simulink model "PoredjenjeLinNelin"  (R2018a)
settings: Solver=VariableStepAuto  StartTime=0.0  StopTime=30  RelTol=1e-3  EnableMultiTasking=on
values from neighbouring files (symbols this model uses):
  a11 = double(subs(diff(f1,wm),[wm id iq u1 mh],[wmn idn iqn u1n mhn]))    [Linearizacija.m]
  a12 = double(subs(diff(f1,id),[wm id iq u1 mh],[wmn idn iqn u1n mhn]))    [Linearizacija.m]
  a13 = double(subs(diff(f1,iq),[wm id iq u1 mh],[wmn idn iqn u1n mhn]))    [Linearizacija.m]
  a21 = double(subs(diff(f2,wm),[wm id iq u1 mh],[wmn idn iqn u1n mhn]))    [Linearizacija.m]
  a22 = double(subs(diff(f2,id),[wm id iq u1 mh],[wmn idn iqn u1n mhn]))    [Linearizacija.m]
  a23 = double(subs(diff(f2,iq),[wm id iq u1 mh],[wmn idn iqn u1n mhn]))    [Linearizacija.m]
  a31 = double(subs(diff(f3,wm),[wm id iq u1 mh],[wmn idn iqn u1n mhn]))    [Linearizacija.m]
  a32 = double(subs(diff(f3,id),[wm id iq u1 mh],[wmn idn iqn u1n mhn]))    [Linearizacija.m]
  a33 = double(subs(diff(f3,iq),[wm id iq u1 mh],[wmn idn iqn u1n mhn]))    [Linearizacija.m]
  b11 = double(subs(diff(f1,u1),[wm id iq u1 mh],[wmn idn iqn u1n mhn]))    [Linearizacija.m]
  b12 = double(subs(diff(f1,mh),[wm id iq u1 mh],[wmn idn iqn u1n mhn]))    [Linearizacija.m]
  b21 = double(subs(diff(f2,u1),[wm id iq u1 mh],[wmn idn iqn u1n mhn]))    [Linearizacija.m]
  b22 = double(subs(diff(f2,mh),[wm id iq u1 mh],[wmn idn iqn u1n mhn]))    [Linearizacija.m]
  b31 = double(subs(diff(f3,u1),[wm id iq u1 mh],[wmn idn iqn u1n mhn]))    [Linearizacija.m]
  b32 = double(subs(diff(f3,mh),[wm id iq u1 mh],[wmn idn iqn u1n mhn]))    [Linearizacija.m]
  Bv = 1.349*10^(-5)    (= 1.349e-05)    [Podaci.m]    (also in Podaci.mat)
  F0 = 0.1717    [Podaci.m]    (also in Podaci.mat)
  idn = Odgovor(2)    [nominale.m]
  iqn = Odgovor(3)    [nominale.m]
  J0 = 3.26*10^-3    (= 0.00326)    [Podaci.m]    (also in Podaci.mat)
  Ls = Ld    (= 0.03682)    [Podaci.m]    (also in Podaci.mat)
  m = 3    [Podaci.m]    (also in Podaci.mat)
  mhn = 0.3    [nominale.m]
  np = 2    [Podaci.m]    (also in Podaci.mat)
  Rs = 16.7    [Podaci.m]    (also in Podaci.mat)
  teta0 = 0    [Podaci.m]    (also in Podaci.mat)
  u1n = Odgovor(1)    [nominale.m]
  wmn = nn*pi/30    (= 314.159265359)    [nominale.m]
settings Model: Creator=Bane  LastModifiedBy=lakim
settings DataIOCC: LimitDataPoints=on
settings OptimizationCC: LifeSpan=inf
settings DebuggingCC: AllowSymbolicDim=off  SFUnexpectedBacktrackingDiag=warning  SFNoUnconditionalDefaultTransitionDiag=warning  SFExecutionAtInitializationDiag=none
settings ModelReferenceCC: PropagateSignalLabelsOutOfModel=off
settings CodeAppCC: StateflowObjectComments=on
settings GRTTargetCC: TargetLangStandard=C89/C90 (ANSI)
settings ConfigComp: CovMetricSettings=dw  CovHtmlReporting=on  CovSaveCumulativeToWorkspaceVar=on  CovSaveSingleToWorkspaceVar=on  CovExternalEMLEnable=off

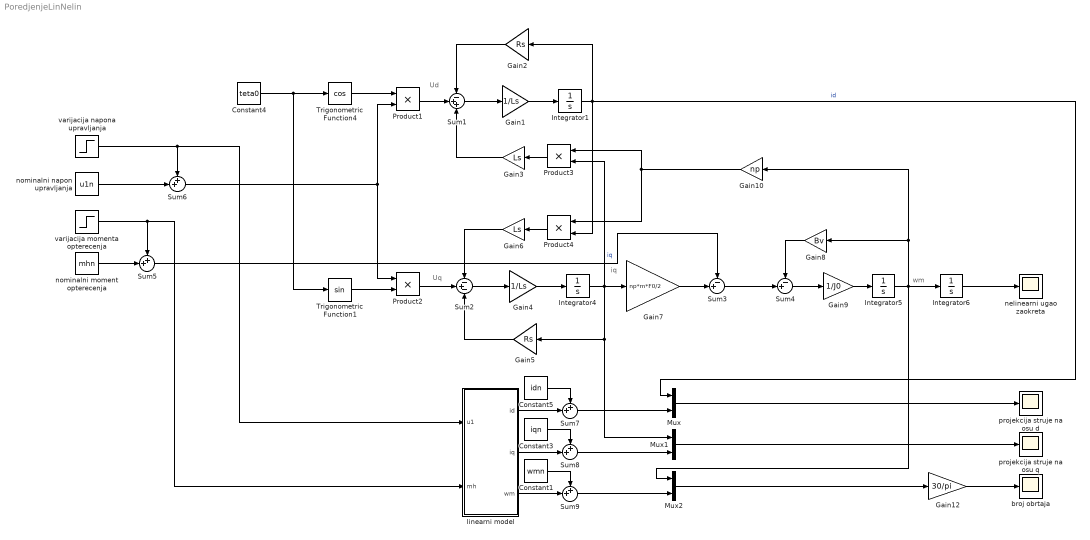
== system PoredjenjeLinNelin ==
  note: Uq
  note: iq
  note: Ud
  note: wm
  " broj obrtaja" : Scope
  Constant1 : Constant  Value=wmn
  Constant3 : Constant  Value=iqn
  Constant4 : Constant  Value=teta0
  Constant5 : Constant  Value=idn
  Gain1 : Gain  Gain=1/Ls
  Gain10 : Gain  Gain=np
  Gain12 : Gain  Gain=30/pi
  Gain2 : Gain  Gain=Rs
  Gain3 : Gain  Gain=Ls
  Gain4 : Gain  Gain=1/Ls
  Gain5 : Gain  Gain=Rs
  Gain6 : Gain  Gain=Ls
  Gain7 : Gain  Gain=np*m*F0/2
  Gain8 : Gain  Gain=Bv
  Gain9 : Gain  Gain=1/J0
  Integrator1 : Integrator  InitialCondition=idn
  Integrator4 : Integrator  InitialCondition=iqn
  Integrator5 : Integrator  InitialCondition=wmn
  Integrator6 : Integrator
  Mux : Mux  Inputs=2
  Mux1 : Mux  Inputs=2
  Mux2 : Mux  Inputs=2
  Product{1..4} (4 alike) : Product
  Sum1 : Sum  Inputs=-++
  Sum2 : Sum  Inputs=-+-
  Sum3 : Sum  Inputs=-+|
  Sum4 : Sum  Inputs=-+|
  Sum{5..9} (5 alike) : Sum  Inputs=++|
  Trigonometric Function1 : Trigonometry
  Trigonometric Function4 : Trigonometry  Operator=cos
  linearni model : Subsystem
  nelinearni ugao zaokreta : Scope
  nominalni moment opterecenja : Constant  Value=mhn
  nominalni napon upravljanja : Constant  Value=u1n
  projekcija struje na osu d : Scope
  projekcija struje na osu q : Scope
  "varijacija momenta opterecenja " : Step  Time=3  After=0.3  SampleTime=0
  varijacija napona upravljanja : Step  Time=0  After=0  SampleTime=0
  wires:
  Gain1/1 -> Integrator1/1
  Integrator1/1 -> Mux/1, Product4/2, Gain2/1  "id"
  Gain2/1 -> Sum1/1
  Sum1/1 -> Gain1/1
  Trigonometric Function1/1 -> Product2/2
  Trigonometric Function4/1 -> Product1/1
  Constant4/1 -> Trigonometric Function1/1, Trigonometric Function4/1
  Product1/1 -> Sum1/2
  Product3/1 -> Gain3/1
  Gain3/1 -> Sum1/3
  Gain4/1 -> Integrator4/1
  Integrator4/1 -> Mux1/1, Gain5/1, Gain7/1, Product3/2  "iq"
  Sum2/1 -> Gain4/1
  Product2/1 -> Sum2/2
  Product4/1 -> Gain6/1
  Gain6/1 -> Sum2/1
  Gain5/1 -> Sum2/3
  Gain9/1 -> Integrator5/1
  Integrator5/1 -> Mux2/1, Integrator6/1, Gain10/1, Gain8/1
  Sum4/1 -> Gain9/1
  Gain8/1 -> Sum4/1
  Gain10/1 -> Product4/1, Product3/1
  Integrator6/1 -> nelinearni ugao zaokreta/1
  Gain7/1 -> Sum3/2
  Sum3/1 -> Sum4/2
  nominalni moment opterecenja/1 -> Sum5/2
  Sum5/1 -> Sum3/1
  "varijacija momenta opterecenja "/1 -> linearni model/2(mh), Sum5/1
  Sum6/1 -> Product2/1, Product1/2
  nominalni napon upravljanja/1 -> Sum6/2
  varijacija napona upravljanja/1 -> Sum6/1, linearni model/1(u1)
  Mux/1 -> projekcija struje na osu d/1
  Mux2/1 -> Gain12/1
  linearni model/1(id) -> Sum7/2
  Sum7/1 -> Mux/2
  linearni model/2(iq) -> Sum8/2
  linearni model/3(wm) -> Sum9/2
  Sum9/1 -> Mux2/2
  Constant5/1 -> Sum7/1
  Constant3/1 -> Sum8/1
  Constant1/1 -> Sum9/1
  Gain12/1 -> " broj obrtaja"/1
  Mux1/1 -> projekcija struje na osu q/1
  Sum8/1 -> Mux1/2

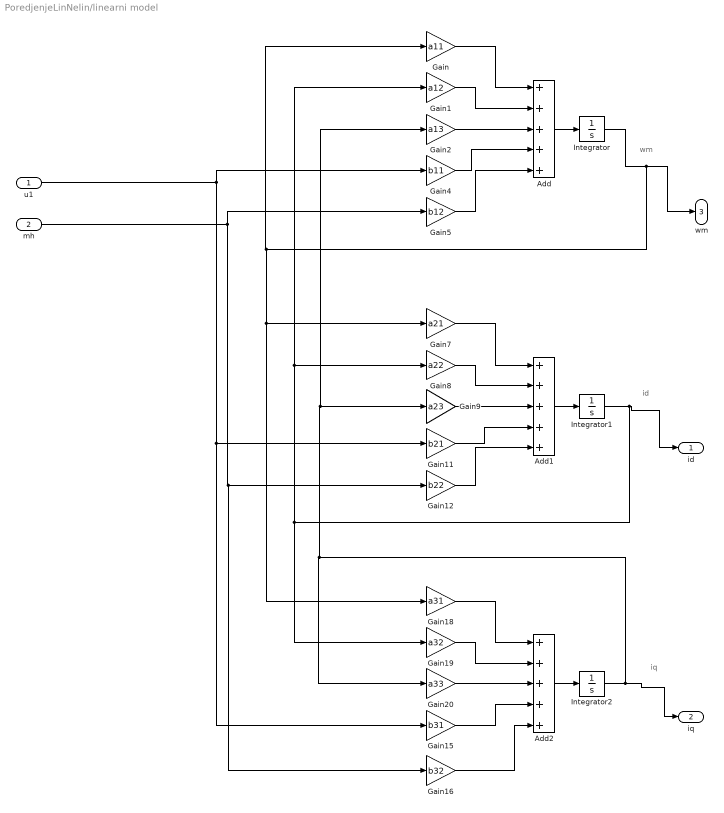
== system PoredjenjeLinNelin/linearni model ==
  note: wm
  note: iq
  note: id
  u1 : Inport
  mh : Inport  Port=2
  Add : Sum  Inputs=+++++
  Add1 : Sum  Inputs=+++++
  Add2 : Sum  Inputs=+++++
  Gain : Gain  Gain=a11
  Gain1 : Gain  Gain=a12
  Gain11 : Gain  Gain=b21
  Gain12 : Gain  Gain=b22
  Gain15 : Gain  Gain=b31
  Gain16 : Gain  Gain=b32
  Gain18 : Gain  Gain=a31
  Gain19 : Gain  Gain=a32
  Gain2 : Gain  Gain=a13
  Gain20 : Gain  Gain=a33
  Gain4 : Gain  Gain=b11
  Gain5 : Gain  Gain=b12
  Gain7 : Gain  Gain=a21
  Gain8 : Gain  Gain=a22
  Gain9 : Gain  Gain=a23
  Integrator : Integrator
  Integrator1 : Integrator
  Integrator2 : Integrator
  id : Outport  VectorParamsAs1DForOutWhenUnconnected=on
  iq : Outport  Port=2  VectorParamsAs1DForOutWhenUnconnected=on
  wm : Outport  Port=3  VectorParamsAs1DForOutWhenUnconnected=on
  wires:
  Gain4/1 -> Add/4
  Gain5/1 -> Add/5
  Gain18/1 -> Add2/1
  Gain2/1 -> Add/3
  Add2/1 -> Integrator2/1
  Integrator1/1 -> Gain19/1, Gain8/1, Gain1/1, id/1
  Gain7/1 -> Add1/1
  Gain9/1 -> Add1/3
  Gain20/1 -> Add2/3
  Gain19/1 -> Add2/2
  Add/1 -> Integrator/1
  Gain/1 -> Add/1
  Gain8/1 -> Add1/2
  Gain1/1 -> Add/2
  Add1/1 -> Integrator1/1
  Integrator2/1 -> Gain2/1, Gain9/1, Gain20/1, iq/1
  Gain15/1 -> Add2/4
  Gain16/1 -> Add2/5
  mh/1 -> Gain16/1, Gain12/1, Gain5/1
  Gain11/1 -> Add1/4
  Gain12/1 -> Add1/5
  Integrator/1 -> Gain18/1, Gain7/1, Gain/1, wm/1
  u1/1 -> Gain4/1, Gain15/1, Gain11/1
